simulink model "ACC"  (R2023b)
settings: Solver=FixedStepAuto  StartTime=0.0  StopTime=inf  RelTol=1e-3
libraries: arduinolib x8
settings Model: ExtModeTrigDuration=2  Creator=SJ  LastModifiedBy=SJ
settings SolverCC: AutoInsertRateTranBlk=on
settings OptimizationCC: EnhancedBackFolding=on  PassReuseOutputArgsAs=Individual arguments  ZeroExternalMemoryAtStartup=off  ZeroInternalMemoryAtStartup=off  MaxStackSize=64  OptimizeBlockOrder=speed  DifferentSizesBufferReuse=on  OptimizationCustomize=off  EfficientTunableParamExpr=on
settings DebuggingCC: MultiTaskDSMMsg=none  ParameterTunabilityLossMsg=error
settings HardwareCC: ProdBitPerInt=16  ProdBitPerPointer=16  ProdBitPerSizeT=16  ProdBitPerPtrDiffT=16  ProdLargestAtomicFloat=None  ProdWordSize=8  ProdHWDeviceType=Atmel->AVR
settings SFSimCC: MATLABDynamicMemAlloc=off
settings RTWCC: Description=Embedded Coder  SystemTargetFile=ert.tlc  HardwareBoard=Arduino Mega 2560  TemplateMakefile=ert_default_tmf  Toolchain=Arduino AVR  BuildConfiguration=Faster Runs
settings CodeAppCC: ForceParamTrailComments=on  IgnoreCustomStorageClasses=off  OperatorAnnotations=on  SimulinkDataObjDesc=on  SFDataObjDesc=on  InsertBlockDesc=on
settings ERTTargetCC: SupportContinuousTime=on  SupportVariableSizeSignals=on  ExtModeTransport=3  ExtModeStaticAlloc=on  ExtModeAutomaticAllocSize=off  ExtModeStaticAllocSize=2048  ExtModeMexFile=ext_xcp  ExtModeIntrfLevel=Level2 - Open

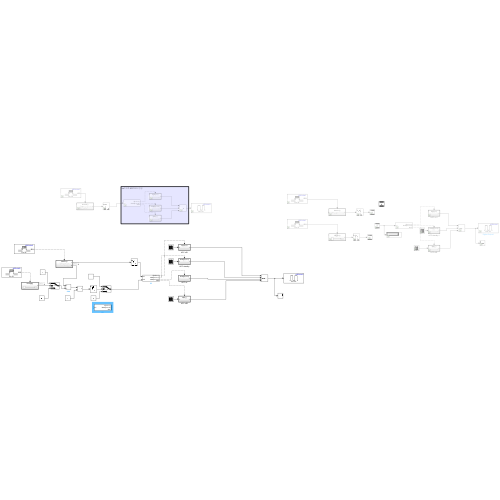
[thumbnail: Simulink's stored preview of the top-level diagram]
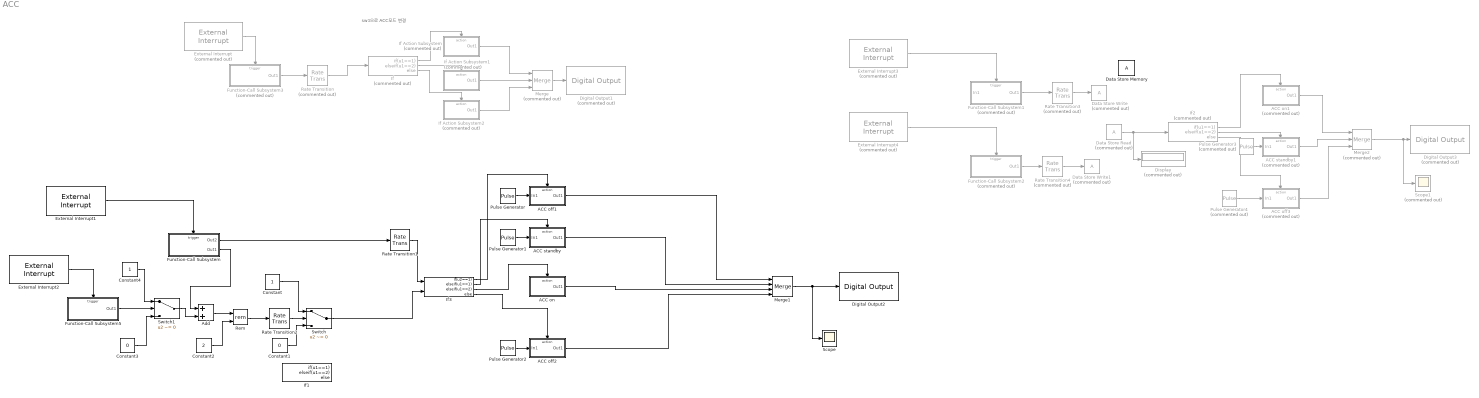
== system ACC ==
  note: sw1으로 ACC모드 변경
  ACC off1 : Subsystem  TreatAsAtomicUnit=on
  ACC off2 : Subsystem  TreatAsAtomicUnit=on
  ACC off3 : Subsystem  Commented=on  TreatAsAtomicUnit=on
  ACC on : Subsystem  TreatAsAtomicUnit=on
  ACC on1 : Subsystem  Commented=on  TreatAsAtomicUnit=on
  ACC standby : Subsystem  TreatAsAtomicUnit=on
  ACC standby1 : Subsystem  Commented=on  TreatAsAtomicUnit=on
  Add : Sum
  Constant : Constant
  Constant1 : Constant  Value=0
  Constant2 : Constant  Value=2
  Constant3 : Constant  Value=0
  Constant4 : Constant
  Data Store Memory : DataStoreMemory  WriteAfterWriteMsg=warning  ShowAdditionalParam=off
  Data Store Read : DataStoreRead  Commented=on  IndexOptions=Index vector (dialog)  Indices=1  OutputSizes=1
  Data Store Write : DataStoreWrite  Commented=on  IndexOptions=Index vector (dialog)  Indices=1  OutputSizes=1
  Data Store Write1 : DataStoreWrite  Commented=on  IndexOptions=Index vector (dialog)  Indices=1  OutputSizes=1
  Digital Output1 : arduinolib/Digital Output  Commented=on  pinNumber=22  Direction=output  blockPlatform=arduino
  Digital Output2 : arduinolib/Digital Output  pinNumber=22  Direction=output  blockPlatform=arduino
  Digital Output3 : arduinolib/Digital Output  Commented=on  pinNumber=22  Direction=output  blockPlatform=arduino
  Display : Display  Commented=on
  External Interrupt : arduinolib/External Interrupt  Commented=on  Pin=20  PullUp=off  Mode=RISING  InterruptSimulationInput=off
  External Interrupt1 : arduinolib/External Interrupt  Pin=20  PullUp=off  Mode=FALLING  InterruptSimulationInput=off
  External Interrupt2 : arduinolib/External Interrupt  Pin=21  PullUp=off  Mode=FALLING  InterruptSimulationInput=off
  External Interrupt3 : arduinolib/External Interrupt  Commented=on  Pin=20  PullUp=off  Mode=FALLING  InterruptSimulationInput=off
  External Interrupt4 : arduinolib/External Interrupt  Commented=on  Pin=21  PullUp=off  Mode=FALLING  InterruptSimulationInput=off
  Function-Call Subsystem : Subsystem  TreatAsAtomicUnit=on
  Function-Call Subsystem1 : Subsystem  Commented=on  TreatAsAtomicUnit=on
  Function-Call Subsystem2 : Subsystem  Commented=on  TreatAsAtomicUnit=on
  Function-Call Subsystem3 : Subsystem  Commented=on  TreatAsAtomicUnit=on
  Function-Call Subsystem5 : Subsystem  TreatAsAtomicUnit=on
  If : If  Commented=on  IfExpression=u1==1  ElseIfExpressions=u1==2
  If Action Subsystem : Subsystem  Commented=on  TreatAsAtomicUnit=on
  If Action Subsystem1 : Subsystem  Commented=on  TreatAsAtomicUnit=on
  If Action Subsystem2 : Subsystem  Commented=on  TreatAsAtomicUnit=on
  If1 : If  IfExpression=u1==1  ElseIfExpressions=u1==2
  If2 : If  Commented=on  IfExpression=u1==1  ElseIfExpressions=u1==2
  If3 : If  NumInputs=2  IfExpression=u2==1  ElseIfExpressions=u1==1,u1==2
  Merge : Merge  Commented=on  Inputs=3
  Merge1 : Merge  Inputs=4
  Merge2 : Merge  Commented=on  Inputs=3
  Pulse Generator : DiscretePulseGenerator  PulseType=Time based  PulseWidth=50
  Pulse Generator1 : DiscretePulseGenerator  PulseType=Time based  Period=0.4  PulseWidth=50
  Pulse Generator2 : DiscretePulseGenerator  PulseType=Time based  PulseWidth=50
  Pulse Generator3 : DiscretePulseGenerator  Commented=on  PulseType=Time based  Amplitude=5  PulseWidth=50
  Pulse Generator4 : DiscretePulseGenerator  Commented=on  PulseType=Time based  PulseWidth=50
  Rate Transition : RateTransition  Commented=on  Deterministic=off
  Rate Transition1 : RateTransition  Deterministic=off  OutPortSampleTime=0.01
  Rate Transition2 : RateTransition  Deterministic=off  OutPortSampleTime=0.01
  Rate Transition3 : RateTransition  Commented=on  Deterministic=off  OutPortSampleTime=0.01
  Rate Transition4 : RateTransition  Commented=on  Deterministic=off  OutPortSampleTime=0.01
  Rem : Math  Operator=rem
  Scope : Scope
  Scope1 : Scope  Commented=on
  Switch : Switch  Criteria=u2 ~= 0  SaturateOnIntegerOverflow=off  InputSameDT=off
  Switch1 : Switch  Criteria=u2 ~= 0  SaturateOnIntegerOverflow=off  InputSameDT=off
  wires:
  External Interrupt/1 -> Function-Call Subsystem3/Trigger
  Function-Call Subsystem3/1(Out1) -> Rate Transition/1
  Merge/1 -> Digital Output1/1
  If Action Subsystem1/1(Out1) -> Merge/2
  If/3 -> If Action Subsystem2/Action
  If/2 -> If Action Subsystem1/Action
  Rate Transition/1 -> If/1
  If/1 -> If Action Subsystem/Action
  If Action Subsystem/1(Out1) -> Merge/1
  If Action Subsystem2/1(Out1) -> Merge/3
  External Interrupt2/1 -> Function-Call Subsystem5/Trigger
  Rate Transition1/1 -> If3/1
  External Interrupt1/1 -> Function-Call Subsystem/Trigger
  Function-Call Subsystem/1(Out2) -> Rate Transition1/1
  Merge1/1 -> Scope/1, Digital Output2/1
  ACC off1/1(Out1) -> Merge1/1
  ACC standby/1(Out1) -> Merge1/2
  ACC on/1(Out1) -> Merge1/3
  External Interrupt4/1 -> Function-Call Subsystem2/Trigger
  External Interrupt3/1 -> Function-Call Subsystem1/Trigger
  If2/1 -> ACC on1/Action
  If2/2 -> ACC standby1/Action
  If2/3 -> ACC off3/Action
  ACC on1/1(Out1) -> Merge2/1
  ACC standby1/1(Out1) -> Merge2/2
  ACC off3/1(Out1) -> Merge2/3
  Merge2/1 -> Scope1/1, Digital Output3/1
  Data Store Read/1 -> Display/1, If2/1
  Function-Call Subsystem1/1(Out1) -> Rate Transition3/1
  Function-Call Subsystem2/1(Out1) -> Rate Transition4/1
  Rate Transition3/1 -> Data Store Write/1
  Rate Transition4/1 -> Data Store Write1/1
  Pulse Generator/1 -> ACC off1/1(In1)
  Pulse Generator1/1 -> ACC standby/1(In1)
  Pulse Generator2/1 -> ACC off2/1(In1)
  Pulse Generator3/1 -> ACC standby1/1(In1)
  Pulse Generator4/1 -> ACC off3/1(In1)
  Switch/1 -> If3/2
  If3/1 -> ACC off1/Action
  If3/2 -> ACC standby/Action
  If3/3 -> ACC on/Action
  If3/4 -> ACC off2/Action
  ACC off2/1(Out1) -> Merge1/4
  Constant/1 -> Switch/1
  Constant1/1 -> Switch/3
  Rate Transition2/1 -> Switch/2
  Function-Call Subsystem/2(Out1) -> Add/1
  Add/1 -> Rem/1
  Constant2/1 -> Rem/2
  Function-Call Subsystem5/1(Out1) -> Switch1/2
  Switch1/1 -> Add/2
  Constant3/1 -> Switch1/3
  Constant4/1 -> Switch1/1
  Rem/1 -> Rate Transition2/1

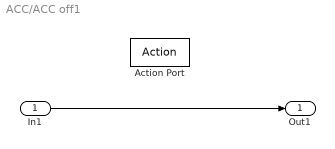
== system ACC/ACC off1 ==
  In1 : Inport
  Action Port : ActionPort  ActionPortLabel=if(u2==1)
  Out1 : Outport
  wires:
  In1/1 -> Out1/1

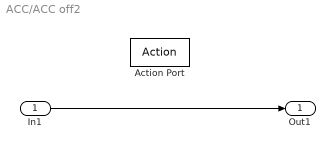
== system ACC/ACC off2 ==
  In1 : Inport
  Action Port : ActionPort  ActionPortLabel=else
  Out1 : Outport
  wires:
  In1/1 -> Out1/1

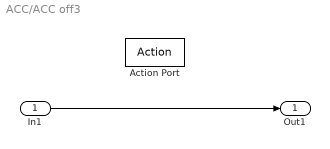
== system ACC/ACC off3 ==
  In1 : Inport
  Action Port : ActionPort  ActionPortLabel=else
  Out1 : Outport
  wires:
  In1/1 -> Out1/1

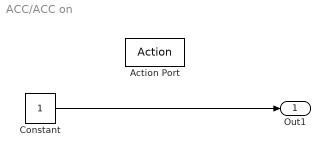
== system ACC/ACC on ==
  Action Port : ActionPort  ActionPortLabel=elseif(u1==2)
  Constant : Constant
  Out1 : Outport
  wires:
  Constant/1 -> Out1/1

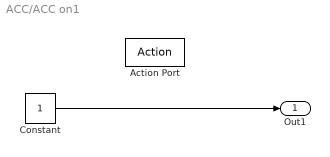
== system ACC/ACC on1 ==
  Action Port : ActionPort  ActionPortLabel=if(u1==1)
  Constant : Constant
  Out1 : Outport
  wires:
  Constant/1 -> Out1/1

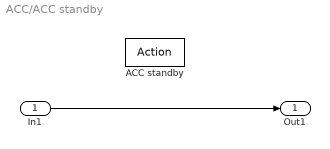
== system ACC/ACC standby ==
  In1 : Inport
  ACC standby : ActionPort  ActionPortLabel=elseif(u1==1)
  Out1 : Outport
  wires:
  In1/1 -> Out1/1

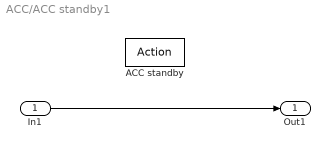
== system ACC/ACC standby1 ==
  In1 : Inport
  ACC standby : ActionPort  ActionPortLabel=elseif(u1==2)
  Out1 : Outport
  wires:
  In1/1 -> Out1/1

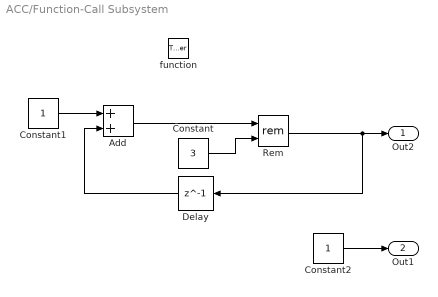
== system ACC/Function-Call Subsystem ==
  function : TriggerPort  TriggerType=function-call  VariantControl=(inherit)
  Add : Sum
  Constant : Constant  Value=3
  Constant1 : Constant
  Constant2 : Constant
  Delay : Delay  DelayLength=1
  Rem : Math  Operator=rem
  Out2 : Outport
  Out1 : Outport  Port=2
  wires:
  Constant/1 -> Rem/2
  Delay/1 -> Add/2
  Add/1 -> Rem/1
  Constant1/1 -> Add/1
  Rem/1 -> Out2/1, Delay/1
  Constant2/1 -> Out1/1

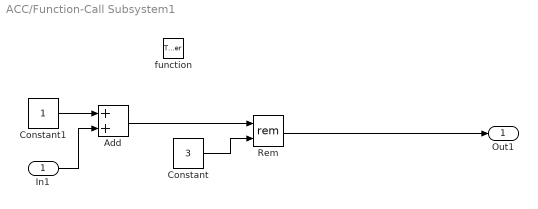
== system ACC/Function-Call Subsystem1 ==
  In1 : Inport
  function : TriggerPort  TriggerType=function-call  VariantControl=(inherit)
  Add : Sum
  Constant : Constant  Value=3
  Constant1 : Constant
  Rem : Math  Operator=rem
  Out1 : Outport
  wires:
  Constant/1 -> Rem/2
  Rem/1 -> Out1/1
  Add/1 -> Rem/1
  Constant1/1 -> Add/1
  In1/1 -> Add/2

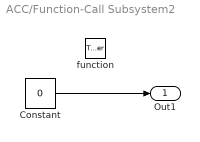
== system ACC/Function-Call Subsystem2 ==
  function : TriggerPort  TriggerType=function-call  VariantControl=(inherit)
  Constant : Constant  Value=0
  Out1 : Outport
  wires:
  Constant/1 -> Out1/1

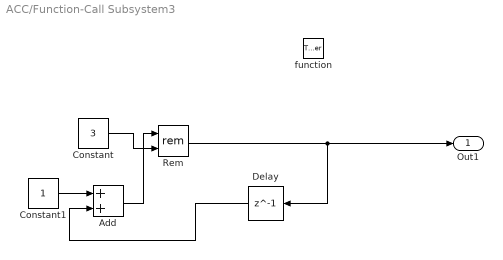
== system ACC/Function-Call Subsystem3 ==
  function : TriggerPort  TriggerType=function-call  VariantControl=(inherit)
  Add : Sum
  Constant : Constant  Value=3
  Constant1 : Constant
  Delay : Delay  DelayLength=1  InitialCondition=0
  Rem : Math  Operator=rem
  Out1 : Outport
  wires:
  Rem/1 -> Delay/1, Out1/1
  Delay/1 -> Add/2
  Constant1/1 -> Add/1
  Constant/1 -> Rem/2
  Add/1 -> Rem/1

== system ACC/Function-Call Subsystem5 ==
  function : TriggerPort  TriggerType=function-call  VariantControl=(inherit)
  Constant : Constant
  Out1 : Outport
  wires:
  Constant/1 -> Out1/1

== system ACC/If Action Subsystem ==
  Action Port : ActionPort  ActionPortLabel=if(u1==1)
  Pulse Generator : DiscretePulseGenerator  PulseType=Time based  Period=0.4  PulseWidth=50
  Out1 : Outport
  wires:
  Pulse Generator/1 -> Out1/1

== system ACC/If Action Subsystem1 ==
  Action Port : ActionPort  ActionPortLabel=elseif(u1==2)
  Constant : Constant
  Out1 : Outport
  wires:
  Constant/1 -> Out1/1

== system ACC/If Action Subsystem2 ==
  Action Port : ActionPort  ActionPortLabel=else
  Constant : Constant  Value=0
  Out1 : Outport
  wires:
  Constant/1 -> Out1/1
